simulink model "PTC_MBDS_ScrollLineWrapAround_Sample"  (R2013a)
settings: Solver=VariableStepDiscrete  StartTime=0.0  StopTime=100  RelTol=1e-3
undefined symbols (not defined in the file): sigbuilder_block
libraries: PTC_MBDS_LIB x2, simulink_extras x1
Description:
  | MBDS example or test model
settings Model: Creator=uid60719  LastModifiedBy=sundeep.tuteja
settings DataIOCC: LimitDataPoints=off  SignalLoggingSaveFormat=ModelDataLogs  SaveOutput=off  SignalLogging=off  SaveTime=off
settings OptimizationCC: ExpressionDepthLimit=2147483647  InitFltsAndDblsToZero=on
settings DebuggingCC: SaveWithParameterizedLinksMsg=none  SignalResolutionControl=TryResolveAllWithWarning  SolverPrmCheckMsg=none  InheritedTsInSrcMsg=none  DiscreteInheritContinuousMsg=none  MultiTaskDSMMsg=warning  MultiTaskCondExecSysMsg=none  FcnCallInpInsideContextMsg=UseLocalSettings  StrictBusMsg=Warning
settings RTWCC: IncludeERTFirstTime=on
settings GRTTargetCC: TargetFcnLib=ansi_tfl_tmw.mat  CombineOutputUpdateFcns=off  GRTInterface=on

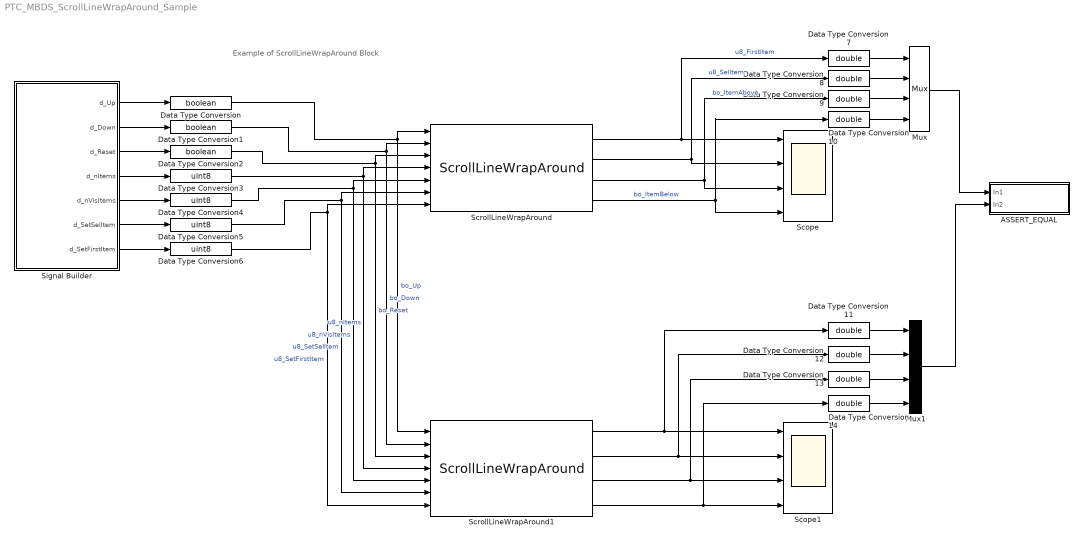
== system PTC_MBDS_ScrollLineWrapAround_Sample ==
  note: Example of ScrollLineWrapAround Block
  ASSERT_EQUAL : Subsystem
  Data Type Conversion : DataTypeConversion  OutDataTypeStr=boolean
      settings: MoveFcn=UpdateBlockSize(gcb);
  Data Type Conversion1 : DataTypeConversion  OutDataTypeStr=boolean
      settings: MoveFcn=UpdateBlockSize(gcb);
  Data Type Conversion2 : DataTypeConversion  OutDataTypeStr=boolean
      settings: MoveFcn=UpdateBlockSize(gcb);
  Data Type Conversion{3..6} (4 alike) : DataTypeConversion  OutDataTypeStr=uint8
      settings: MoveFcn=UpdateBlockSize(gcb);
  Data Type Conversion{7..14} (8 alike) : DataTypeConversion  OutDataTypeStr=double
  Mux : Mux
  Mux1 : Mux
  Scope : Scope  NumInputPorts=4
      settings: YMin=-5~-5~-5~-5  YMax=5~5~5~5
  Scope1 : Scope  NumInputPorts=4
      settings: YMin=-5~-5~-5~-5  YMax=5~5~5~5
  ScrollLineWrapAround : PTC_MBDS_LIB/MBDS Standard Library/Extended Operations/HMI/ScrollLineWrapAround  PTC_MBDS_BlockVersion=5.32  PTC_BlockType=PTC_MBDS_ScrollLineWrapAround
  ScrollLineWrapAround1 : PTC_MBDS_LIB/MBDS Standard Library/Extended Operations/HMI/ScrollLineWrapAround  PTC_MBDS_BlockVersion=5.32  PTC_BlockType=PTC_MBDS_ScrollLineWrapAround
  Signal Builder : Subsystem  Tag=STV Subsys  LoadFcn=sigbuilder_block('load');  StartFcn=sigbuilder_block('start');  StopFcn=sigbuilder_block('stop');  ClipboardFcn=sigbuilder_block('clipboard');  mask(Sigbuilder block){}
      mask help: Create and generate interchangeable groups of signals whose waveforms are piecewise linear.
      mask init:
      | if ~strcmp(get_param(bdroot(gcbh),'SimulationStatus'),'stopped') tuvar = sigbuilder_block('maskInit'); end
      settings: CopyFcn=sigbuilder_block('copy');  DeleteFcn=sigbuilder_block('delete');  ModelCloseFcn=sigbuilder_block('modelClose');  PreSaveFcn=sigbuilder_block('preSave');  PauseFcn=sigbuilder_block('pause')  ContinueFcn=sigbuilder_block('continue')  NameChangeFcn=sigbuilder_block('namechange');  OpenFcn=sigbuilder_block('open',[1040.25 116.25 472.5 441 ]);  CloseFcn=sigbuilder_block('close');
      mask Display: plot(0,0,100,100,[10,10,40,40,10],[80,20,20,80,80],[40,10],[50,50], [40,27,10],[65,72,56],[40,25,25,10],[28,28,43,43]);
  wires:
  Signal Builder/1(d_Up) -> Data Type Conversion/1
  Signal Builder/2(d_Down) -> Data Type Conversion1/1
  Signal Builder/3(d_Reset) -> Data Type Conversion2/1
  Signal Builder/4(d_nItems) -> Data Type Conversion3/1
  Data Type Conversion/1 -> ScrollLineWrapAround1/1, ScrollLineWrapAround/1  "bo_Up"
  Data Type Conversion1/1 -> ScrollLineWrapAround1/2, ScrollLineWrapAround/2  "bo_Down"
  Data Type Conversion2/1 -> ScrollLineWrapAround1/3, ScrollLineWrapAround/3  "bo_Reset"
  Data Type Conversion3/1 -> ScrollLineWrapAround1/4, ScrollLineWrapAround/4  "u8_nItems"
  Signal Builder/5(d_nVisItems) -> Data Type Conversion4/1
  Signal Builder/6(d_SetSelItem) -> Data Type Conversion5/1
  Signal Builder/7(d_SetFirstItem) -> Data Type Conversion6/1
  Data Type Conversion4/1 -> ScrollLineWrapAround1/5, ScrollLineWrapAround/5  "u8_nVisItems"
  Data Type Conversion5/1 -> ScrollLineWrapAround1/6, ScrollLineWrapAround/6  "u8_SetSelItem"
  Data Type Conversion6/1 -> ScrollLineWrapAround1/7, ScrollLineWrapAround/7  "u8_SetFirstItem"
  ScrollLineWrapAround/1 -> Data Type Conversion7/1, Scope/1  "u8_FirstItem"
  ScrollLineWrapAround/2 -> Scope/2, Data Type Conversion8/1  "u8_SelItem"
  ScrollLineWrapAround/3 -> Scope/3, Data Type Conversion9/1  "bo_ItemAbove"
  ScrollLineWrapAround/4 -> Scope/4, Data Type Conversion10/1  "bo_ItemBelow"
  ScrollLineWrapAround1/3 -> Data Type Conversion13/1, Scope1/3
  ScrollLineWrapAround1/4 -> Data Type Conversion14/1, Scope1/4
  ScrollLineWrapAround1/1 -> Data Type Conversion11/1, Scope1/1
  ScrollLineWrapAround1/2 -> Data Type Conversion12/1, Scope1/2
  Mux/1 -> ASSERT_EQUAL/1(In1)
  Mux1/1 -> ASSERT_EQUAL/2(In2)
  Data Type Conversion7/1 -> Mux/1
  Data Type Conversion8/1 -> Mux/2
  Data Type Conversion9/1 -> Mux/3
  Data Type Conversion10/1 -> Mux/4
  Data Type Conversion11/1 -> Mux1/1
  Data Type Conversion12/1 -> Mux1/2
  Data Type Conversion13/1 -> Mux1/3
  Data Type Conversion14/1 -> Mux1/4

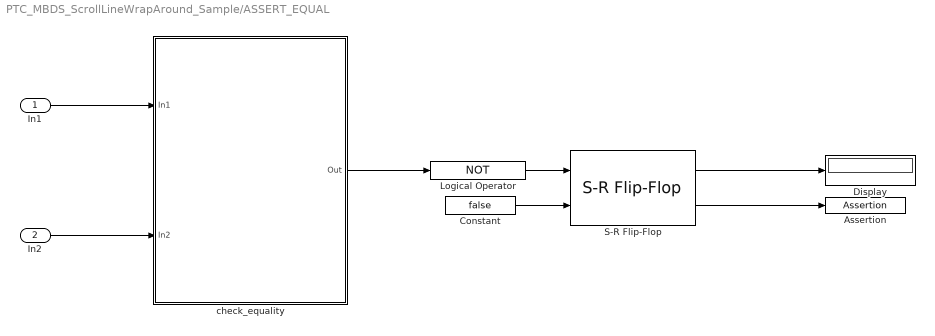
== system PTC_MBDS_ScrollLineWrapAround_Sample/ASSERT_EQUAL ==
  In1 : Inport
  In2 : Inport  Port=2
  Assertion : Assertion
  Constant : Constant  Value=false
  Display : Display
  Logical Operator : Logic  Operator=NOT  AllPortsSameDT=off  OutDataTypeStr=boolean
  S-R Flip-Flop : simulink_extras/Flip Flops/S-R Flip-Flop  initial_condition=0
  check_equality : MATLAB Function  TreatAsAtomicUnit=on
  wires:
  S-R Flip-Flop/1 -> Display/1
  check_equality/1(Out) -> Logical Operator/1
  Constant/1 -> S-R Flip-Flop/2
  S-R Flip-Flop/2 -> Assertion/1
  In2/1 -> check_equality/2(In2)
  In1/1 -> check_equality/1(In1)
  Logical Operator/1 -> S-R Flip-Flop/1

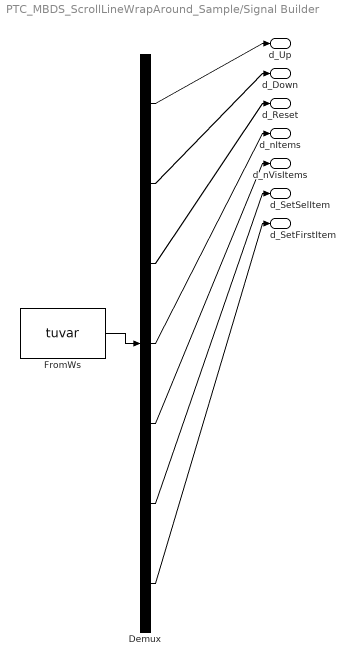
== system PTC_MBDS_ScrollLineWrapAround_Sample/Signal Builder ==
  Demux : Demux  Tag=STV Demux  Outputs=7
  FromWs : FromWorkspace  Tag=STV FromWs  VariableName=tuvar  SampleTime=0
      SigBuilderData=|
      | common.afterFinalStr = 'Extrapolate'
      | common.sampleTime = 0
      | dataSet(1).timeRange = [0 10]
      | dataSet(1).name = 'TC1'
      | dataSet(2).timeRange = [0 10]
      | dataSet(2).name = 'TC2'
      | dataSet(3).timeRange = [0 10]
      | dataSet(3).name = 'TC3'
      | dataSet(4).timeRange = [0 10]
      | dataSet(4).name = 'TC4'
      | dataSet(5).timeRange = [0 10]
      | dataSet(5).name = 'TC5'
      | dataSet(6).timeRange = [0 10]
      | dataSet(6).name = 'TC6'
      | sbobj.Groups(1).Name = 'TC1'
      | sbobj.Groups(1).Signals(1).Name = 'd_Up'
      | sbobj.Groups(1).Signals(1).XData = [0 5.4 5.4 5.8 5.8 6 6 6.4 6.4 6.6 6.6 7 7 7.2 7.2 7.6 7.6 7.8 7.8 8.2 8.2 8.4 8.4 8.8 8.8 9 9 9.4 9.4 9.6 9.6 10]
      | sbobj.Groups(1).Signals(1).YData = [0 0 1 1 0 0 1 1 0 0 1 1 0 0 1 1 0 0 1 1 0 0 1 1 0 0 1 1 0 0 1 1]
      | sbobj.Groups(1).Signals(2).Name = 'd_Down'
      | sbobj.Groups(1).Signals(2).XData = [0 0.6 0.6 1 1 1.2 1.2 1.6 1.6 1.8 1.8 2.2 2.2 2.4 2.4 2.8 2.8 3 3 3.4 3.4 3.6 3.6 4 4 4.2 4.2 4.6 4.6 4.8 4.8 5.2 5.2 10]
      | sbobj.Groups(1).Signals(2).YData = [0 0 1 1 0 0 1 1 0 0 1 1 0 0 1 1 0 0 1 1 0 0 1 1 0 0 1 1 0 0 1 1 0 0]
      | sbobj.Groups(1).Signals(3).Name = 'd_Reset'
      | sbobj.Groups(1).Signals(3).XData = [0 10]
      | sbobj.Groups(1).Signals(3).YData = [0 0]
      | sbobj.Groups(1).Signals(4).Name = 'd_nItems'
      | sbobj.Groups(1).Signals(4).XData = [0 10]
      | sbobj.Groups(1).Signals(4).YData = [6 6]
      | sbobj.Groups(1).Signals(5).Name = 'd_nVisItems'
      | sbobj.Groups(1).Signals(5).XData = [0 10]
      | sbobj.Groups(1).Signals(5).YData = [3 3]
      | sbobj.Groups(1).Signals(6).Name = 'd_SetSelItem'
      | sbobj.Groups(1).Signals(6).XData = [0 10]
      | sbobj.Groups(1).Signals(6).YData = [1 1]
      | sbobj.Groups(1).Signals(7).Name = 'd_SetFirstItem'
      | sbobj.Groups(1).Signals(7).XData = [0 10]
      | sbobj.Groups(1).Signals(7).YData = [0 0]
      | sbobj.Groups(2).Name = 'TC2'
      | sbobj.Groups(2).Signals(1).Name = 'd_Up'
      | sbobj.Groups(2).Signals(1).XData = [0 5.4 5.4 5.8 5.8 6 6 6.4 6.4 6.6 6.6 7 7 7.2 7.2 7.6 7.6 7.8 7.8 8.2 8.2 8.4 8.4 8.8 8.8 9 9 9.4 9.4 9.6 9.6 10]
      | sbobj.Groups(2).Signals(1).YData = [0 0 1 1 0 0 1 1 0 0 1 1 0 0 1 1 0 0 1 1 0 0 1 1 0 0 1 1 0 0 1 1]
      | sbobj.Groups(2).Signals(2).Name = 'd_Down'
      | sbobj.Groups(2).Signals(2).XData = [0 0.6 0.6 1 1 1.2 1.2 1.6 1.6 1.8 1.8 2.2 2.2 2.4 2.4 2.8 2.8 3 3 3.4 3.4 3.6 3.6 4 4 4.2 4.2 4.6 4.6 4.8 4.8 5.2 5.2 10]
      | sbobj.Groups(2).Signals(2).YData = [0 0 1 1 0 0 1 1 0 0 1 1 0 0 1 1 0 0 1 1 0 0 1 1 0 0 1 1 0 0 1 1 0 0]
      | sbobj.Groups(2).Signals(3).Name = 'd_Reset'
      | sbobj.Groups(2).Signals(3).XData = [0 10]
      | sbobj.Groups(2).Signals(3).YData = [0 0]
      | sbobj.Groups(2).Signals(4).Name = 'd_nItems'
      | sbobj.Groups(2).Signals(4).XData = [0 10]
      | sbobj.Groups(2).Signals(4).YData = [6 6]
      | sbobj.Groups(2).Signals(5).Name = 'd_nVisItems'
      | sbobj.Groups(2).Signals(5).XData = [0 10]
      | sbobj.Groups(2).Signals(5).YData = [2 2]
      | sbobj.Groups(2).Signals(6).Name = 'd_SetSelItem'
      | sbobj.Groups(2).Signals(6).XData = [0 10]
      | sbobj.Groups(2).Signals(6).YData = [1 1]
      | sbobj.Groups(2).Signals(7).Name = 'd_SetFirstItem'
      | sbobj.Groups(2).Signals(7).XData = [0 10]
      | sbobj.Groups(2).Signals(7).YData = [0 0]
      | sbobj.Groups(3).Name = 'TC3'
      | sbobj.Groups(3).Signals(1).Name = 'd_Up'
      | sbobj.Groups(3).Signals(1).XData = [0 10]
      | sbobj.Groups(3).Signals(1).YData = [0 0]
      | sbobj.Groups(3).Signals(2).Name = 'd_Down'
      | sbobj.Groups(3).Signals(2).XData = [0 0.6 0.6 1 1 1.2 1.2 1.6 1.6 1.8 1.8 2.2 2.2 2.4 2.4 2.8 2.8 3 3 3.4 3.4 3.6 3.6 4 4 4.2 4.2 4.6 4.6 4.8 4.8 5.2 5.2 5.4 5.4 5.8 5.8 6 6 6.4 6.4 6.6 6.6 7 7 7.2 7.2 7.6 7.6 7.8 7.8 8.2 8.2 8.4 8.4 8.8 8.8 9 9 9.4 9.4 9.6 9.6 10]
      | sbobj.Groups(3).Signals(2).YData = [0 0 1 1 0 0 1 1 0 0 1 1 0 0 1 1 0 0 1 1 0 0 1 1 0 0 1 1 0 0 1 1 0 0 1 1 0 0 1 1 0 0 1 1 0 0 1 1 0 0 1 1 0 0 1 1 0 0 1 1 0 0 1 1]
      | sbobj.Groups(3).Signals(3).Name = 'd_Reset'
      | sbobj.Groups(3).Signals(3).XData = [0 10]
      | sbobj.Groups(3).Signals(3).YData = [0 0]
      | sbobj.Groups(3).Signals(4).Name = 'd_nItems'
      | sbobj.Groups(3).Signals(4).XData = [0 10]
      | sbobj.Groups(3).Signals(4).YData = [6 6]
      | sbobj.Groups(3).Signals(5).Name = 'd_nVisItems'
      | sbobj.Groups(3).Signals(5).XData = [0 10]
      | sbobj.Groups(3).Signals(5).YData = [6 6]
      | sbobj.Groups(3).Signals(6).Name = 'd_SetSelItem'
      | sbobj.Groups(3).Signals(6).XData = [0 10]
      | sbobj.Groups(3).Signals(6).YData = [0 0]
      | sbobj.Groups(3).Signals(7).Name = 'd_SetFirstItem'
      | sbobj.Groups(3).Signals(7).XData = [0 10]
      | sbobj.Groups(3).Signals(7).YData = [0 0]
      | sbobj.Groups(4).Name = 'TC4'
      | sbobj.Groups(4).Signals(1).Name = 'd_Up'
      | sbobj.Groups(4).Signals(1).XData = [0 10]
      | sbobj.Groups(4).Signals(1).YData = [0 0]
      | sbobj.Groups(4).Signals(2).Name = 'd_Down'
      | sbobj.Groups(4).Signals(2).XData = [0 0.6 0.6 1 1 1.2 1.2 1.6 1.6 1.8 1.8 2.2 2.2 2.4 2.4 2.8 2.8 3 3 3.4 3.4 3.6 3.6 4 4 4.2 4.2 4.6 4.6 4.8 4.8 5.2 5.2 5.4 5.4 5.8 5.8 6 6 6.4 6.4 6.6 6.6 7 7 7.2 7.2 7.6 7.6 7.8 7.8 8.2 8.2 8.4 8.4 8.8 8.8 9 9 9.4 9.4 9.6 9.6 10]
      | sbobj.Groups(4).Signals(2).YData = [0 0 1 1 0 0 1 1 0 0 1 1 0 0 1 1 0 0 1 1 0 0 1 1 0 0 1 1 0 0 1 1 0 0 1 1 0 0 1 1 0 0 1 1 0 0 1 1 0 0 1 1 0 0 1 1 0 0 1 1 0 0 1 1]
      | sbobj.Groups(4).Signals(3).Name = 'd_Reset'
      | sbobj.Groups(4).Signals(3).XData = [0 10]
      | sbobj.Groups(4).Signals(3).YData = [0 0]
      | sbobj.Groups(4).Signals(4).Name = 'd_nItems'
      | sbobj.Groups(4).Signals(4).XData = [0 10]
      | sbobj.Groups(4).Signals(4).YData = [6 6]
      | sbobj.Groups(4).Signals(5).Name = 'd_nVisItems'
      | sbobj.Groups(4).Signals(5).XData = [0 10]
      | sbobj.Groups(4).Signals(5).YData = [0 0]
      | sbobj.Groups(4).Signals(6).Name = 'd_SetSelItem'
      | sbobj.Groups(4).Signals(6).XData = [0 10]
      | sbobj.Groups(4).Signals(6).YData = [0 0]
      | sbobj.Groups(4).Signals(7).Name = 'd_SetFirstItem'
      | sbobj.Groups(4).Signals(7).XData = [0 10]
      | sbobj.Groups(4).Signals(7).YData = [0 0]
      | sbobj.Groups(5).Name = 'TC5'
      | sbobj.Groups(5).Signals(1).Name = 'd_Up'
      | sbobj.Groups(5).Signals(1).XData = [0 10]
      | sbobj.Groups(5).Signals(1).YData = [0 0]
      | sbobj.Groups(5).Signals(2).Name = 'd_Down'
      | sbobj.Groups(5).Signals(2).XData = [0 0.6 0.6 1 1 1.2 1.2 1.6 1.6 1.8 1.8 2.2 2.2 2.4 2.4 2.8 2.8 3 3 3.4 3.4 3.6 3.6 4 4 4.2 4.2 4.6 4.6 4.8 4.8 5.2 5.2 5.4 5.4 5.8 5.8 6 6 6.4 6.4 6.6 6.6 7 7 7.2 7.2 7.6 7.6 7.8 7.8 8.2 8.2 8.4 8.4 8.8 8.8 9 9 9.4 9.4 9.6 9.6 10]
      | sbobj.Groups(5).Signals(2).YData = [0 0 1 1 0 0 1 1 0 0 1 1 0 0 1 1 0 0 1 1 0 0 1 1 0 0 1 1 0 0 1 1 0 0 1 1 0 0 1 1 0 0 1 1 0 0 1 1 0 0 1 1 0 0 1 1 0 0 1 1 0 0 1 1]
      | sbobj.Groups(5).Signals(3).Name = 'd_Reset'
      | sbobj.Groups(5).Signals(3).XData = [0 1.8 1.8 2 2 3.6 3.6 3.8 3.8 5.4 5.4 5.6 5.6 10]
      | sbobj.Groups(5).Signals(3).YData = [0 0 1 1 0 0 1 1 0 0 1 1 0 0]
      | sbobj.Groups(5).Signals(4).Name = 'd_nItems'
      | sbobj.Groups(5).Signals(4).XData = [0 10]
      | sbobj.Groups(5).Signals(4).YData = [6 6]
      | sbobj.Groups(5).Signals(5).Name = 'd_nVisItems'
      | sbobj.Groups(5).Signals(5).XData = [0 10]
      | sbobj.Groups(5).Signals(5).YData = [3 3]
      | sbobj.Groups(5).Signals(6).Name = 'd_SetSelItem'
      | sbobj.Groups(5).Signals(6).XData = [0 3.6 3.6 10]
      | sbobj.Groups(5).Signals(6).YData = [0 0 1 1]
      | sbobj.Groups(5).Signals(7).Name = 'd_SetFirstItem'
      | sbobj.Groups(5).Signals(7).XData = [0 5.4 5.4 10]
      | sbobj.Groups(5).Signals(7).YData = [0 0 3 3]
      | sbobj.Groups(6).Name = 'TC6'
      | sbobj.Groups(6).Signals(1).Name = 'd_Up'
      | sbobj.Groups(6).Signals(1).XData = [0 10]
      | sbobj.Groups(6).Signals(1).YData = [0 0]
      | sbobj.Groups(6).Signals(2).Name = 'd_Down'
      | sbobj.Groups(6).Signals(2).XData = [0 0.6 0.6 1 1 1.2 1.2 1.6 1.6 1.8 1.8 2.2 2.2 2.4 2.4 2.8 2.8 3 3 3.4 3.4 3.6 3.6 4 4 4.2 4.2 4.6 4.6 4.8 4.8 5.2 5.2 5.4 5.4 5.8 5.8 6 6 6.4 6.4 6.6 6.6 7 7 7.2 7.2 7.6 7.6 7.8 7.8 8.2 8.2 8.4 8.4 8.8 8.8 9 9 9.4 9.4 9.6 9.6 10]
      | sbobj.Groups(6).Signals(2).YData = [0 0 1 1 0 0 1 1 0 0 1 1 0 0 1 1 0 0 1 1 0 0 1 1 0 0 1 1 0 0 1 1 0 0 1 1 0 0 1 1 0 0 1 1 0 0 1 1 0 0 1 1 0 0 1 1 0 0 1 1 0 0 1 1]
      | sbobj.Groups(6).Signals(3).Name = 'd_Reset'
      | sbobj.Groups(6).Signals(3).XData = [0 10]
      | sbobj.Groups(6).Signals(3).YData = [0 0]
      | sbobj.Groups(6).Signals(4).Name = 'd_nItems'
      | sbobj.Groups(6).Signals(4).XData = [0 10]
      | sbobj.Groups(6).Signals(4).YData = [6 6]
      | sbobj.Groups(6).Signals(5).Name = 'd_nVisItems'
      | sbobj.Groups(6).Signals(5).XData = [0 10]
      | sbobj.Groups(6).Signals(5).YData = [0 0]
      | sbobj.Groups(6).Signals(6).Name = 'd_SetSelItem'
      | sbobj.Groups(6).Signals(6).XData = [0 10]
      | sbobj.Groups(6).Signals(6).YData = [0 0]
      | sbobj.Groups(6).Signals(7).Name = 'd_SetFirstItem'
      | sbobj.Groups(6).Signals(7).XData = [0 10]
      | sbobj.Groups(6).Signals(7).YData = [0 0]
  d_Up : Outport  Tag=STV Outport
  d_Down : Outport  Tag=STV Outport  Port=2
  d_Reset : Outport  Tag=STV Outport  Port=3
  d_nItems : Outport  Tag=STV Outport  Port=4
  d_nVisItems : Outport  Tag=STV Outport  Port=5
  d_SetSelItem : Outport  Tag=STV Outport  Port=6
  d_SetFirstItem : Outport  Tag=STV Outport  Port=7
  wires:
  Demux/7 -> d_SetFirstItem/1
  Demux/6 -> d_SetSelItem/1
  Demux/5 -> d_nVisItems/1
  Demux/4 -> d_nItems/1
  Demux/3 -> d_Reset/1
  Demux/2 -> d_Down/1
  Demux/1 -> d_Up/1
  FromWs/1 -> Demux/1

== matlab function PTC_MBDS_ScrollLineWrapAround_Sample/ASSERT_EQUAL/check_equality ==
  data: In1 input; Out output; In2 input
function Out = check_equality(In1, In2)
%#codegen

Out = isequaln(In1, In2);

end
